simulink model "TechnoEconomicMicrogrid"  (R2025a)
settings: Solver=VariableStepAuto  StartTime=0.0  StopTime=tPeriod-1  FixedStep=sampleTime  RelTol=1e-3
PostLoadFcn:
  | TechnoEconomicAnalysisInput
undefined symbols (not defined in the file): batteryProfile, batteryStorage, DiscIntNeverNeededParam, EMS, generatorProfile, generatorSet, line, loadForecast, mainGrid, optimizationInterval, optimizationMode, solarForecast, solarPV, windFarm, windForecast, windPowerEst
libraries: ee_lib x11, fl_lib x9, simulink x5, eeGeneralControl x4, nesl_utility x3, simulink_extras x1
(part 2 of 2)

== matlab function TechnoEconomicMicrogrid/Microgrid Controller/Supervisory Control/MATLAB Function2 ==
  data: bessPref input; generatorLoading input; flag input; PRefBattery output; index input; PRefGenerator output; optimizationInterval input
function [PRefBattery,PRefGenerator] = arrayOutput(bessPref,generatorLoading,flag,index,optimizationInterval)

    % Ensure the input array is a column vector
    bessPref = bessPref(:);
    generatorLoading = generatorLoading(:);

    % % Determine the index based on the current time (1-based indexing)
    % index = floor(currentTime) + 1;

    % Ensure the index does not exceed the length of the array
    
    if flag < 1
         PRefBattery = bessPref(1);
         PRefGenerator = generatorLoading(1);
    else
          index = rem(index+1,optimizationInterval);
          if index < 1
              index = 1;
          end
          PRefBattery = bessPref(index);
          PRefGenerator = generatorLoading(index);
    end
end

== stateflow chart TechnoEconomicMicrogrid/Microgrid Controller/Supervisory Control/Rule Based EMS/Wind ==
  (default) -> (junction 19) : % Battery Reference Generation
  (junction 62) -> (junction 83)
  (junction 19) -> (junction 62) [order 1] : [batterySOCFlag == true]
  (junction 83) -> (junction 85)
  (junction 19) -> (junction 18) [order 6]
  (junction 45) -> (junction 55) [order 3]
  (junction 19) -> (junction 20) [order 2] : [bessReserve > 0 && bessReserve > forecast*rating && bessPRef>=0]
  (junction 20) -> (junction 77) [order 2] : {bessPRef = batteryMaxPower;
      | bessReserveCal = batteryMaxPower;}
  (junction 19) -> (junction 45) [order 5] : [bessPRef < 0]
  (junction 19) -> (junction 21) [order 3] : [bessReserve > 0 && bessReserve < forecast*rating && bessPRef>=0]
  (junction 19) -> (junction 22) [order 4] : [forecast*rating <= 0 && bessPRef>=0 ]
  (junction 20) -> (junction 75) [order 1] : [forecast*rating+batteryForecast < batteryMaxPower]
  (junction 77) -> (junction 79)
  (junction 45) -> (junction 51) [order 2] : [forecast*rating >= 0 && forecast*rating < bessReserve]
  (junction 21) -> (junction 73)
  (junction 51) -> (junction 53) : {bessPRef = forecast*rating;
      | bessReserveCal = batteryMaxPower;}
  (junction 45) -> (junction 47) [order 1] : [forecast*rating > bessReserve]
  (junction 73) -> (junction 23) : {bessPRef = batteryMaxPower;
      | bessReserveCal = batteryMaxPower;
      | gridPower = loadForecast-bessPRef-sourceForecast*sourceRating-generatorForecast*generatorRating;
      | }
  (junction 75) -> (junction 28) : {bessPRef = forecast*rating+batteryForecast;
      | bessReserveCal = batteryMaxPower;}
  (junction 49) -> (junction 22)
  (junction 87) -> (junction 22)
  (junction 22) -> (junction 24) : {gridPower = loadForecast-sourceForecast*sourceRating-generatorForecast*generatorRating;}
  (junction 47) -> (junction 49) : {bessPRef = batteryMaxPower;
      | bessReserveCal = batteryMaxPower;}
  (junction 28) -> (junction 79)
  (junction 24) -> (junction 67) [order 2]
  (junction 23) -> (junction 67) [order 2]
  (junction 24) -> (junction 26) [order 1] : [gridPower > gridPowerMax]
  (junction 23) -> (junction 25) [order 1] : [gridPower > gridPowerMax]{excessLoad = gridPowerMax-gridPower;}
  (junction 26) -> (junction 29) : {loadShedding = true;}
  (junction 25) -> (junction 27) : {loadShedding = true;}
  (junction 85) -> (junction 87)
  data: batteryForecast input double; generatorForecast input double; loadForecast input double; bessPRef output double; bessReserve input double; batteryMaxPower input double; excessLoad data_store_memory; gridPowerMax input double; loadShedding output boolean; batterySOCFlag input boolean; sourceForecast input double; rating input double; forecast input double; sourceRating input double; gridPower local double; charging input; bessReserveCal output double; generatorRating input double

== matlab function TechnoEconomicMicrogrid/Microgrid Controller/Supervisory Control/Optimization Based EMS/Reference Generation ==
  data: batteryPower input; pRefBattery output; wind input; solar input; generatorPower input; load input; flag input; batterySOC input; pRefGenerator output; loadShedding output; time input; gridCost parameter; fuelCost parameter; batteryMinSOC parameter; batteryMaxSOC parameter; gridMinPower parameter; gridMaxPower parameter; batteryMinPower parameter; batteryMaxPower parameter; batteryEnergyRating parameter; windRating parameter; generatorRating parameter; solarRating parameter; fuelType input double
 function [pRefBattery,pRefGenerator,loadShedding] = fcn(batteryPower,wind,solar,generatorPower,load,flag,batterySOC,time,gridCost, fuelCost, batteryMinSOC, batteryMaxSOC, gridMinPower, gridMaxPower, batteryMinPower, batteryMaxPower, batteryEnergyRating, windRating, generatorRating, solarRating, fuelType)
% Get the specific element
optimizationInterval = 6;
loadForecast = load(time+1:time+optimizationInterval);
solarForecast = solar(time+1:time+optimizationInterval);
windForecast = wind(time+1:time+optimizationInterval);
generatorForecast = generatorPower(time+1:time+optimizationInterval);
batteryForecast = batteryPower(time+1:time+optimizationInterval);

% Battery constraints
% Initialize the constraints
battery.minPower = batteryMinPower;
battery.maxPower = batteryMaxPower;
battery.minSOC = batteryMinSOC;
battery.maxSOC = batteryMaxSOC;
battery.forecast = batteryForecast;
battery.initialSOC = batterySOC;
battery.energyRating = batteryEnergyRating;

% Grid constraints
% Initialize the constraints
grid.maxPower = gridMaxPower;
grid.minPower = gridMinPower;
grid.cost = gridCost;


% Generator constraint
generator.rating = generatorRating;
generator.forecast = generatorForecast;
generator.fuelCost = fuelCost;
generator.fuel = fuelType;

if flag == 1
    renewableForecast = solarRating*solarForecast;
elseif flag == 2
    renewableForecast = windRating*windForecast;
else
    renewableForecast = 0;
end

optimizationSteps = optimizationInterval;
timeInterval = 1;

% Declare function (contains linprog) as extrinsic
 coder.extrinsic('onlineOptimization');
% 
pRefBattery = ones(length(batteryForecast),1);
pRefGenerator = ones(length(batteryForecast),1);
loadShedding = 0;

[pRefBattery,pRefGenerator,loadShedding] = onlineOptimization(grid,battery,loadForecast,renewableForecast,generator,optimizationSteps,timeInterval);
end
